simulink model "sampleModel1517_sub"  (R2023a)
settings: Solver=VariableStepAuto  StartTime=0.0  StopTime=10.0  RelTol=1e-3
libraries: hdlsllib x3, simulink x1
settings Model: Creator=user1  LastModifiedBy=user1
settings OptimizationCC: BlockReduction=off  ConditionallyExecuteInputs=off

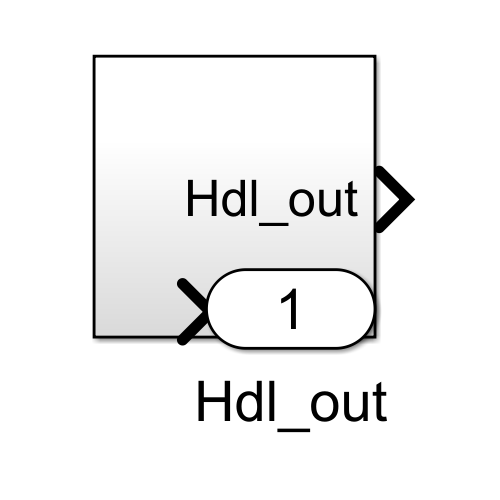
[thumbnail: Simulink's stored preview of the top-level diagram]
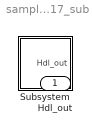
== system sampleModel1517_sub ==
  Subsystem : Subsystem
  Hdl_out : Outport  OutDataTypeStr=uint8

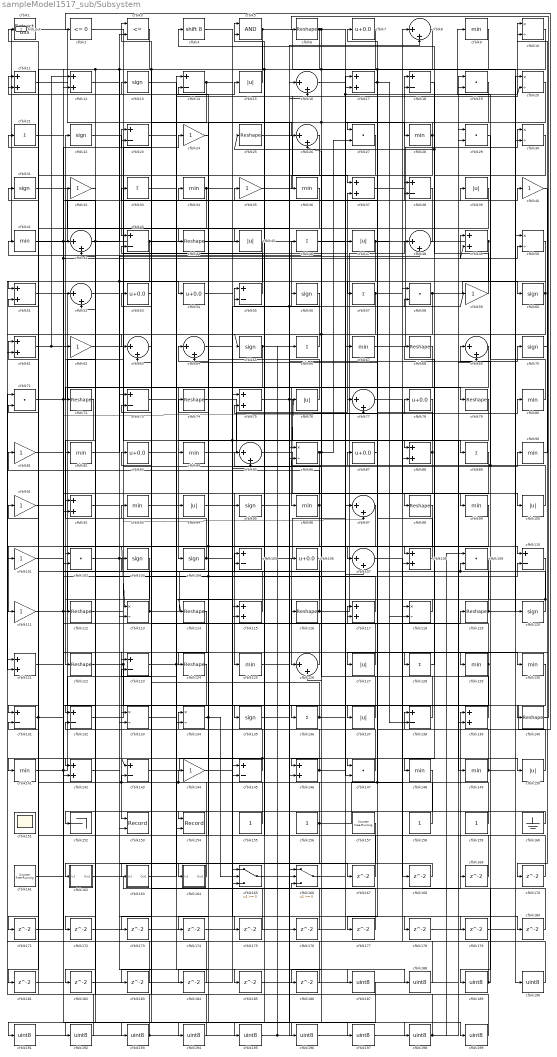
== system sampleModel1517_sub/Subsystem ==
  cfblk1 : simulink/Logic and Bit Operations/Extract Bits  bitsToExtract=Upper half  numBits=8  bitIdxRange=[0 7]  outScalingMode=Preserve fixed-point scaling
      settings: LibrarySourceBlock=|
      | hdlsllib/Logic and Bit
      | Operations/Extract Bits
  cfblk{10,20,30,50,86,113,118,133..134} (9 alike) : Product  Inputs=*/  OutDataTypeStr=uint8  RndMeth=Zero  SaturateOnIntegerOverflow=on
  cfblk{15,39,45,47,76,94,100,127,137,150} (10 alike) : Abs  OutDataTypeStr=uint8  SaturateOnIntegerOverflow=off
  cfblk{24,32,35,40,59,62,81,91,101,111,144} (11 alike) : Gain  OutDataTypeStr=uint8
  cfblk{19,27,29,58,71,102,109,147} (8 alike) : DotProduct  OutDataTypeStr=uint8
  cfblk{13,22,31,56,60,65,70,95,103..104,120,135} (12 alike) : Signum
  cfblk{14,18,23,38,43,55,73,105,110,123,131..132,138,143,145} (15 alike) : Sum  Inputs=+-  OutDataTypeStr=uint8
  cfblk{7,53..54,78,83,87,106} (7 alike) : Bias  Bias=0.0  SaturateOnIntegerOverflow=off
  cfblk{8,16,26,42,48,52,63..64,69,77,85,97,107,126} (14 alike) : Sum  Inputs=|++  OutDataTypeStr=uint8
  cfblk{11..12,17,37,49,51,61,75,88,92,108,115,117,121,139,142,146} (17 alike) : Sum  OutDataTypeStr=uint8
  cfblk{6,25,44,68,72,74,79,98,112,114,116,119,122,124,140} (15 alike) : Reshape
  cfblk{9,28,34,36,41,67,80,82,84,90,93,96,99,125,129..130,141,148..149} (19 alike) : MinMax  OutDataTypeStr=uint8
  cfblk{21,33,46,57,66,89,128,136} (8 alike) : Sum  Inputs=+  OutDataTypeStr=uint8
  cfblk151 : Scope
      settings: Floating=on
  cfblk152 : Terminator
  cfblk153 : Record  FileSettingsInternal="{\"entries\":[{\"content\":{\"excelSettings\":{\"content\":{},\"type\":\"Streamout.ExcelSettings\"}},\"type\":\"Streamout.FileSettingStorage\",\"uuid\":\"\"}],\"packageUris\":[\"http:\\/\\/schema.mathworks.com\\/mf0\\/streamout_blocks\\/R2020a\"],\"version\":\"1.0\"}"  Layout=[1 1]  SignalsInternal="{\"entries\":[{\"content\":{\"signals\":[{\"content\":{\"blockPath\":[],\"dimensions\":[1],\"domain\":\"\",\"lineColor\":\"#a2142f\",\"plots\":[1],\"port\":1,\"signalID\":23250,\"signalName\":\"cfblk114\"},\"type\":\"RecordBlkView.Signal\",\"uuid\":\"\"},{\"content\":{\"blockPath\":[],\"dimensions\":[1],\"domain\":\"\",\"lineColor\":\"#139fff\",\"plots\":[1],\"port\":2,\"signalID\":23253,\"signalName\":\"cfblk27\"},\"type\":\"RecordBlkView.Signal\",\"uuid\":\"\"}]},\"type\":\"RecordBlkView.InputSignals\",\"uuid\":\"\"}],\"packageUris\":[\"http:\\/\\/schema.mathworks.com\\/mf0\\/streamout_blocks\\/R2020a\"],\"version\":\"1.0\"}"  VisualizationBindings="{\"xyplotplugin\":{\"info\":[{\"series\":[{\"bindingParametersList\":[{\"parameter\":\"X-Axis\",\"signalID\":23250,\"signalName\":\"cfblk114\"},{\"parameter\":\"Y-Axis\",\"signalID\":23253,\"signalName\":\"cfblk27\"}],\"seriesID\":45701}],\"subplotID\":1}]}}"  CompatibilityTag=XY  st=-1
  cfblk154 : Record  FileSettingsInternal="{\"entries\":[{\"content\":{\"excelSettings\":{\"content\":{},\"type\":\"Streamout.ExcelSettings\"}},\"type\":\"Streamout.FileSettingStorage\",\"uuid\":\"\"}],\"packageUris\":[\"http:\\/\\/schema.mathworks.com\\/mf0\\/streamout_blocks\\/R2020a\"],\"version\":\"1.0\"}"  Layout=[1 1]  SignalsInternal="{\"entries\":[{\"content\":{\"signals\":[{\"content\":{\"blockPath\":[],\"dimensions\":[1],\"domain\":\"\",\"lineColor\":\"#a2142f\",\"plots\":[1],\"port\":1,\"signalID\":23242,\"signalName\":\"cfblk160\"},\"type\":\"RecordBlkView.Signal\",\"uuid\":\"\"},{\"content\":{\"blockPath\":[],\"dimensions\":[1],\"domain\":\"\",\"lineColor\":\"#139fff\",\"plots\":[1],\"port\":2,\"signalID\":23245,\"signalName\":\"cfblk129\"},\"type\":\"RecordBlkView.Signal\",\"uuid\":\"\"}]},\"type\":\"RecordBlkView.InputSignals\",\"uuid\":\"\"}],\"packageUris\":[\"http:\\/\\/schema.mathworks.com\\/mf0\\/streamout_blocks\\/R2020a\"],\"version\":\"1.0\"}"  VisualizationBindings="{\"xyplotplugin\":{\"info\":[{\"series\":[{\"bindingParametersList\":[{\"parameter\":\"X-Axis\",\"signalID\":23242,\"signalName\":\"cfblk160\"},{\"parameter\":\"Y-Axis\",\"signalID\":23245,\"signalName\":\"cfblk129\"}],\"seriesID\":44595}],\"subplotID\":1}]}}"  CompatibilityTag=XY  st=-1
  cfblk{155..156,158..159} (4 alike) : Constant  OutDataTypeStr=uint8  SampleTime=-1
  cfblk157 : hdlsllib/Sources/Counter Free-Running  NumBits=16  tsamp=-1
  cfblk160 : Ground
  cfblk161 : hdlsllib/Sources/Counter Free-Running  NumBits=16  tsamp=-1
  cfblk162 : Subsystem
      settings: LibrarySourceBlock=|
      | hdlsllib/Ports &
      | Subsystems/Subsystem
  cfblk163 : Subsystem
      settings: LibrarySourceBlock=|
      | hdlsllib/Ports &
      | Subsystems/Subsystem
  cfblk164 : Subsystem
      settings: LibrarySourceBlock=|
      | hdlsllib/Ports &
      | Subsystems/Subsystem
  cfblk165 : Switch  OutDataTypeStr=uint8  SaturateOnIntegerOverflow=off  InputSameDT=off
  cfblk166 : Switch  OutDataTypeStr=uint8  SaturateOnIntegerOverflow=off  InputSameDT=off
  cfblk{167..186} (20 alike) : Delay  SampleTime=1
  cfblk{187..199} (13 alike) : DataTypeConversion  OutDataTypeStr=uint8  SaturateOnIntegerOverflow=off  RndMeth=Floor
  cfblk2 : hdlsllib/Logic and Bit Operations/Compare To Zero  relop=<=  OutDataTypeStr=uint8
  cfblk3 : RelationalOperator  Operator=<=  OutDataTypeStr=boolean  InputSameDT=off
  cfblk4 : ArithShift  BitShiftNumber=8
  cfblk5 : Logic  AllPortsSameDT=off  OutDataTypeStr=boolean
  Hdl_out : Outport  OutDataTypeStr=uint8
  wires:
  cfblk20/1 -> cfblk196/1, cfblk184/1
  cfblk51/1 -> cfblk96/1
  cfblk96/1 -> cfblk81/1, cfblk113/1, cfblk141/1
  cfblk59/1 -> cfblk4/1, cfblk25/1
  cfblk138/1 -> cfblk41/1
  cfblk132/1 -> cfblk90/1
  cfblk145/1 -> cfblk143/1, cfblk134/1
  cfblk53/1 -> cfblk193/1
  cfblk40/1 -> cfblk127/1
  cfblk80/1 -> cfblk9/1
  cfblk67/1 -> cfblk30/1
  cfblk102/1 -> cfblk185/1, cfblk24/1
  cfblk165/1 -> cfblk16/1
  cfblk61/1 -> cfblk12/1, cfblk137/1
  cfblk72/1 -> cfblk122/1
  cfblk97/1 -> cfblk174/1, cfblk133/1
  cfblk25/1 -> cfblk37/1
  cfblk104/1 -> cfblk56/1, cfblk22/1
  cfblk79/1 -> cfblk146/1
  cfblk98/1 -> cfblk111/1
  cfblk85/1 -> cfblk100/1
  cfblk146/1 -> cfblk49/1, cfblk62/1
  cfblk89/1 -> cfblk164/1(In1)
  cfblk116/1 -> cfblk21/1, cfblk48/1
  cfblk84/1 -> cfblk37/2
  cfblk94/1 -> cfblk125/1
  cfblk6/1 -> cfblk142/2, cfblk186/1, cfblk67/1
  cfblk30/1 -> cfblk98/1
  cfblk112/1 -> cfblk47/1
  cfblk5/1 -> cfblk145/2, cfblk120/1
  cfblk114/1 -> cfblk153/1
  cfblk147/1 -> cfblk83/1
  cfblk26/1 -> cfblk101/1
  cfblk2/1 -> cfblk88/1
  cfblk162/1(Out1) -> cfblk139/1
  cfblk141/1 -> cfblk105/2, cfblk14/1
  cfblk108/1 -> cfblk87/1
  cfblk19/1 -> cfblk195/1
  cfblk95/1 -> cfblk70/1
  cfblk106/1 -> cfblk135/1
  cfblk62/1 -> cfblk97/1
  cfblk143/1 -> cfblk147/1
  cfblk46/1 -> cfblk129/1
  cfblk69/1 -> cfblk104/1
  cfblk49/1 -> Hdl_out/1, cfblk133/2, cfblk102/1
  cfblk119/1 -> cfblk50/1, cfblk75/2, cfblk109/2
  cfblk44/1 -> cfblk88/2, cfblk165/1
  cfblk86/1 -> cfblk124/1, cfblk26/2, cfblk27/2
  cfblk164/1(Out1) -> cfblk73/2, cfblk144/1
  cfblk18/1 -> cfblk148/1
  cfblk22/1 -> cfblk43/1
  cfblk105/1 -> cfblk80/1
  cfblk54/1 -> cfblk145/1
  cfblk60/1 -> cfblk51/1, cfblk65/1, cfblk136/1
  cfblk134/1 -> cfblk165/2, cfblk34/1
  cfblk99/1 -> cfblk147/2
  cfblk122/1 -> cfblk176/1, cfblk97/2
  cfblk41/1 -> cfblk140/1, cfblk35/1
  cfblk139/1 -> cfblk85/1
  cfblk129/1 -> cfblk154/2, cfblk74/1
  cfblk81/1 -> cfblk42/1
  cfblk68/1 -> cfblk132/1
  cfblk35/1 -> cfblk10/1
  cfblk101/1 -> cfblk23/1
  cfblk48/1 -> cfblk45/1
  cfblk90/1 -> cfblk10/2
  cfblk23/1 -> cfblk94/1
  cfblk103/1 -> cfblk162/1(In1)
  cfblk24/1 -> cfblk44/1
  cfblk109/1 -> cfblk126/1
  cfblk87/1 -> cfblk7/1
  cfblk78/1 -> cfblk84/1
  cfblk123/1 -> cfblk178/1, cfblk128/1
  cfblk50/1 -> cfblk107/1
  cfblk8/1 -> cfblk142/1
  cfblk160/1 -> cfblk154/1
  cfblk140/1 -> cfblk6/1
  cfblk55/1 -> cfblk3/1
  cfblk156/1 -> cfblk165/3, cfblk108/2, cfblk55/1
  cfblk82/1 -> cfblk48/2
  cfblk166/1 -> cfblk17/2
  cfblk71/1 -> cfblk77/2, cfblk50/2
  cfblk110/1 -> cfblk126/2
  cfblk47/1 -> cfblk138/2, cfblk131/1
  cfblk37/1 -> cfblk18/1
  cfblk127/1 -> cfblk106/1
  cfblk57/1 -> cfblk121/2, cfblk8/1
  cfblk31/1 -> cfblk146/2
  cfblk111/1 -> cfblk123/1, cfblk78/1
  cfblk14/1 -> cfblk26/1, cfblk163/1(In1)
  cfblk34/1 -> cfblk171/1, cfblk108/1
  cfblk118/1 -> cfblk116/1
  cfblk77/1 -> cfblk99/1
  cfblk58/1 -> cfblk82/1, cfblk60/1
  cfblk126/1 -> cfblk23/2
  cfblk17/1 -> cfblk118/2, cfblk57/1
  cfblk3/1 -> cfblk181/1, cfblk92/1
  cfblk73/1 -> cfblk18/2
  cfblk148/1 -> cfblk152/1
  cfblk65/1 -> cfblk150/1, cfblk134/2
  cfblk158/1 -> cfblk117/1, cfblk61/1
  cfblk91/1 -> cfblk198/1
  cfblk21/1 -> cfblk110/1
  cfblk28/1 -> cfblk63/2, cfblk27/1
  cfblk120/1 -> cfblk114/1, cfblk33/1
  cfblk161/1 -> cfblk49/2, cfblk40/1
  cfblk155/1 -> cfblk143/2, cfblk31/1
  cfblk83/1 -> cfblk39/1
  cfblk9/1 -> cfblk52/2, cfblk95/1
  cfblk38/1 -> cfblk63/1
  cfblk15/1 -> cfblk5/1
  cfblk76/1 -> cfblk11/1
  cfblk159/1 -> cfblk77/1
  cfblk66/1 -> cfblk46/1
  cfblk136/1 -> cfblk103/1, cfblk107/2
  cfblk117/1 -> cfblk42/2, cfblk64/1
  cfblk63/1 -> cfblk13/1
  cfblk137/1 -> cfblk105/1
  cfblk144/1 -> cfblk58/2
  cfblk115/1 -> cfblk32/1
  cfblk45/1 -> cfblk61/2
  cfblk75/1 -> cfblk89/1, cfblk38/2, cfblk59/1
  cfblk1/1 -> cfblk166/1
  cfblk121/1 -> cfblk119/1
  cfblk11/1 -> cfblk73/1
  cfblk29/1 -> cfblk189/1
  cfblk56/1 -> cfblk55/2
  cfblk13/1 -> cfblk115/2
  cfblk113/1 -> cfblk38/1, cfblk11/2
  cfblk7/1 -> cfblk12/2, cfblk36/1
  cfblk149/1 -> cfblk117/2, cfblk30/2
  cfblk88/1 -> cfblk92/2, cfblk64/2
  cfblk128/1 -> cfblk68/1
  cfblk12/1 -> cfblk79/1
  cfblk74/1 -> cfblk149/1
  cfblk163/1(Out1) -> cfblk15/1
  cfblk16/1 -> cfblk20/2, cfblk28/1
  cfblk43/1 -> cfblk130/1, cfblk112/1
  cfblk100/1 -> cfblk69/1, cfblk76/1
  cfblk52/1 -> cfblk54/1
  cfblk10/1 -> cfblk177/1, cfblk173/1, cfblk113/2, cfblk72/1
  cfblk130/1 -> cfblk2/1
  cfblk27/1 -> cfblk153/2
  cfblk4/1 -> cfblk139/2
  cfblk131/1 -> cfblk51/2, cfblk110/2
  cfblk150/1 -> cfblk138/1
  cfblk125/1 -> cfblk8/2
  cfblk39/1 -> cfblk102/2
  cfblk42/1 -> cfblk182/1, cfblk3/2
  cfblk142/1 -> cfblk167/1
  cfblk167/1 -> cfblk1/1
  cfblk107/1 -> cfblk168/1
  cfblk168/1 -> cfblk166/2
  cfblk169/1 -> cfblk5/2
  cfblk70/1 -> cfblk170/1
  cfblk170/1 -> cfblk14/2
  cfblk171/1 -> cfblk52/1
  cfblk32/1 -> cfblk172/1
  cfblk172/1 -> cfblk115/1
  cfblk173/1 -> cfblk16/2
  cfblk174/1 -> cfblk17/1
  cfblk133/1 -> cfblk175/1
  cfblk175/1 -> cfblk75/1
  cfblk176/1 -> cfblk123/2
  cfblk177/1 -> cfblk166/3
  cfblk178/1 -> cfblk20/1
  cfblk64/1 -> cfblk179/1
  cfblk92/1 -> cfblk180/1
  cfblk180/1 -> cfblk58/1
  cfblk182/1 -> cfblk85/2
  cfblk124/1 -> cfblk183/1
  cfblk183/1 -> cfblk121/1
  cfblk184/1 -> cfblk131/2
  cfblk185/1 -> cfblk69/2
  cfblk186/1 -> cfblk43/2
  cfblk93/1 -> cfblk187/1
  cfblk33/1 -> cfblk188/1
  cfblk188/1 -> cfblk93/1
  cfblk189/1 -> cfblk118/1, cfblk169/1
  cfblk179/1 -> cfblk190/1
  cfblk190/1 -> cfblk29/1
  cfblk187/1 -> cfblk191/1
  cfblk191/1 -> cfblk29/2
  cfblk157/1 -> cfblk192/1
  cfblk192/1 -> cfblk71/2
  cfblk193/1 -> cfblk71/1, cfblk86/2
  cfblk36/1 -> cfblk194/1
  cfblk194/1 -> cfblk53/1
  cfblk195/1 -> cfblk66/1, cfblk86/1
  cfblk196/1 -> cfblk19/1
  cfblk181/1 -> cfblk197/1
  cfblk197/1 -> cfblk19/2
  cfblk198/1 -> cfblk109/1, cfblk132/2
  cfblk135/1 -> cfblk199/1
  cfblk199/1 -> cfblk91/1

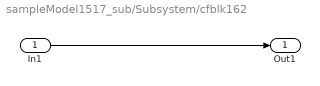
== system sampleModel1517_sub/Subsystem/cfblk162 ==
  In1 : Inport
  Out1 : Outport
  wires:
  In1/1 -> Out1/1

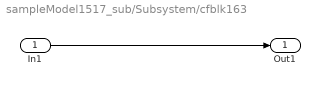
== system sampleModel1517_sub/Subsystem/cfblk163 ==
  In1 : Inport
  Out1 : Outport
  wires:
  In1/1 -> Out1/1

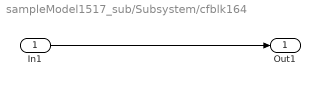
== system sampleModel1517_sub/Subsystem/cfblk164 ==
  In1 : Inport
  Out1 : Outport
  wires:
  In1/1 -> Out1/1
